simulink model "modele6git"  (R2024a)
settings: Solver=VariableStepAuto  StartTime=0.0  StopTime=20  RelTol=1e-6
values from neighbouring files (symbols this model uses):
  A_L = 1    [etablissement_variables.m]
  A_S = 3    [etablissement_variables.m]
  ampli_ent = 1    [etablissement_variables.m]
  C_x = 0.2    [etablissement_variables.m]
  Cte_1 = 10    [etablissement_variables.m]
  Cte_2 = 1.9    [etablissement_variables.m]
  Cte_3 = 1    [etablissement_variables.m]
  Cte_4 = 0.97    [etablissement_variables.m]
  d_f = 1    [etablissement_variables.m]
  d_r = 1    [etablissement_variables.m]
  EPSILON = 1e-9    (= 1e-09)    [etablissement_variables.m]
  f = 0.1    [etablissement_variables.m]
  freq_ent = 0.8    [etablissement_variables.m]
  g = 9.81    [etablissement_variables.m]
  h = 0.4    [etablissement_variables.m]
  Iz = 500    [etablissement_variables.m]
  J = mr/2*R.^2    [etablissement_variables.m]
  L = l_r+l_f    (= 2.9)    [etablissement_variables.m]
  l_f = 1.7    [etablissement_variables.m]
  l_r = 1.2    [etablissement_variables.m]
  M = 400    [etablissement_variables.m]
  R = [0.52 0.52 0.52 0.52]    [etablissement_variables.m]
  rho = 1    [etablissement_variables.m]
undefined symbols (not defined in the file or in its folder): angle_moy, calcul_adherence, calcul_delta, calcul_forceaero, calcul_forces, calcul_lambda, calcul_moteur, calcul_N, calcul_normevitesseroue, calcul_omega, calcul_retourvitesse, calcul_rotaroute, calcul_slipangle, calcul_vitessesroues, check_zeros_1, check_zeros_4, check_zeros_8, eqpfd, projection
libraries: simulink x8, cstblocks x4, spsTriangleGeneratorLib x3, embmathops x1, slpidlib x1
settings Model: SnapshotBufferSize=100  SnapshotInterval=1  Creator=TP-EEA  LastModifiedBy=TP-EEA
settings DebuggingCC: IgnoredZcDiagnostic=none

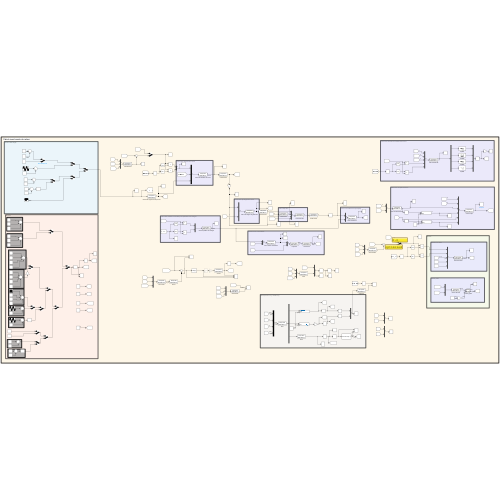
[thumbnail: Simulink's stored preview of the top-level diagram]
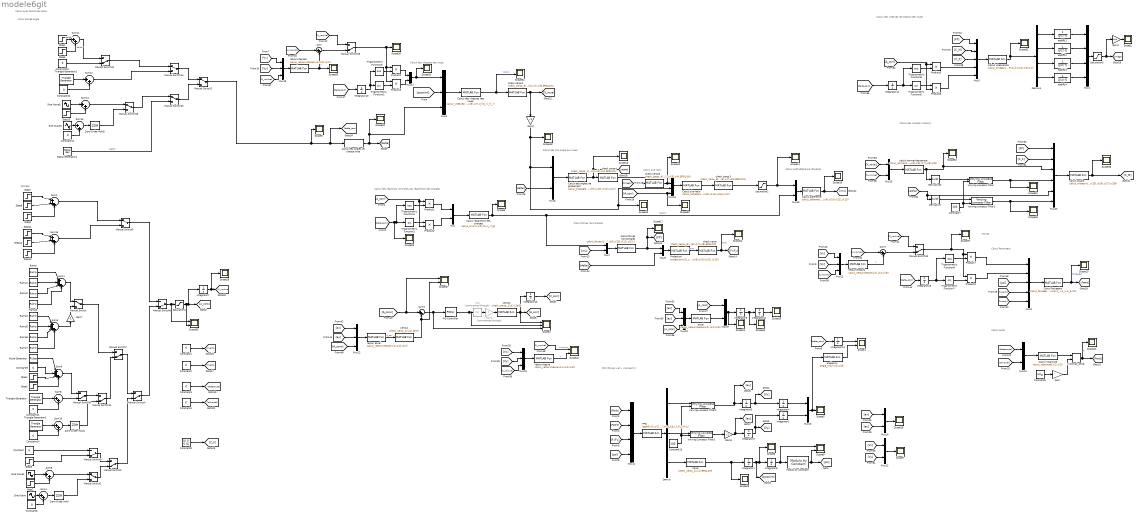
== system modele6git ==
  note: Calcul avec boucle de retour
  note: Calcul des vitesses des roues
  note: Entrées
  note: Choix entrée angle
  note: Calcul des vitesses de rotation des roues
  note: PFD (forces x et y, moment z)
  note: Calcul poids
  note: Calcul des slip-angle aux roues
  note: Calcul coef adhérence (Pacejka)
  note: Calcul slip-ratio
  note: Calcul des réactions normales par répartition des charges
  note: Calcul forces horizontales
  note: Forces
  note: Calcul force aéro
  note: Calcul des couples moteurs
  Abs : Abs  Commented=through  SaturateOnIntegerOverflow=off
  Calcul adhérence : MATLABFcn  MATLABFcn=calcul_adherence(u(1),u(2),u(3),u(4),u(5),u(6),u(7),u(8),Cte_1,Cte_2,Cte_3,Cte_4,u(9),u(10),u(11),u(12))  OutputDimensions=4*2
  Calcul des angles de chaque roue : MATLABFcn  MATLABFcn=calcul_delta(u,L,d_f)  OutputDimensions=4
  Calcul des angles de glissement : MATLABFcn  MATLABFcn=calcul_slipangle(u(1),u(2),u(3),u(4),u(5),u(6),u(7),u(8),u(9),u(10),u(11),u(12))  OutputDimensions=4
  Calcul des vitesses des roues : MATLABFcn  MATLABFcn=calcul_vitessesroues(u(1),u(2),u(3),u(4),u(5),u(6),u(7),d_f,d_r,l_f,l_r)  OutputDimensions=8
  Calcul forceaéro : MATLABFcn  MATLABFcn=calcul_forceaero(u(1),u(2),u(3),u(4),u(5),C_x,A_L,A_S,rho)  OutputDimensions=2
  Calcul forces horizontales : MATLABFcn  MATLABFcn=calcul_forces(u(1),u(2),u(3),u(4),u(5),u(6),u(7),u(8),u(9),u(10),u(11),u(12))  OutputDimensions=4*2
  Calcul rotaroute : MATLABFcn  MATLABFcn=calcul_rotaroute(u(1),u(2))  OutputDimensions=[3 3]  Output1D=off
  Calcul répartition des charges : MATLABFcn  MATLABFcn=calcul_N(u(1),u(2),M,L,l_r,h,g)  OutputDimensions=4
  Calcul slip-ratio : MATLABFcn  MATLABFcn=calcul_lambda(u(1),u(2),u(3),u(4),R(1),R(2),R(3),R(4),u(5),u(6),u(7),u(8),u(9),u(11),u(13),u(15),u(10),u(12),u(14),u(16),u(17))  OutputDimensions=4*2
  Calcul vitesserota : MATLABFcn  MATLABFcn=calcul_omega(u(1),u(2),u(3),u(4),u(5),u(6),u(7),u(8),u(9),u(10),u(11),u(12),u(13),u(14),u(15),u(16),u(17),u(18),R(1),R(2),R(3),R(4),J(1),J(2),J(3),J(4))  OutputDimensions=4
  Constant{,1..4,6,9..12,14..15} (12 alike) : Constant  Value=0
  Constant13 : Constant  Value=100  VectorParams1D=off
  Constant5 : Constant  Value=M*g  VectorParams1D=off
  Constant7 : Constant  Value=100  VectorParams1D=off
  Constant8 : Constant  Value=[0 0 0 0]
  Demux : Demux  Outputs=3
  Demux1 : Demux
  Derivative : Derivative
  Derivative2 : Derivative
  Gain : Gain  Gain=[0 0 1]'
  Gain1 : Gain  Gain=30/pi
  Gain2 : Gain  Gain=-1
  Gain3 : Gain  Gain=-1
  Gain7 : Gain  Gain=-1
  Gain8 : Gain  Commented=through  Gain=-1
  Integrator{1..7,9..15} (14 alike) : Integrator
  Manual Switch{,1..2,5,13..14,16} (7 alike) : ManualSwitch
  Manual Switch{3..4,6..12,15} (10 alike) : ManualSwitch  CurrentSetting=0
  Modulo by Constant : embmathops/Modulo by Constant  Denominator=2*pi  SimulateUsing=Code generation
      settings: LibrarySourceBlock=embeddedMathLib/Modulo by Constant
  Mux{,6..8,10,12..14,16..17,25,37} (12 alike) : Mux  Inputs=2
  Mux1 : Mux
  Mux11 : Mux
  Mux15 : Mux
  Mux{2,18..22} (6 alike) : Mux  Inputs=3
  Mux23 : Mux  Inputs=6
  Mux5 : Mux  Inputs=5
  Mux9 : Mux  Inputs=5
  PFD : MATLABFcn  MATLABFcn=eqpfd(u(1),u(2),u(4),u(5),u(6),u(7),u(8),u(9),u(10),u(11),u(12),u(13),u(14),d_f,d_r,l_f,l_r,M,Iz)  OutputDimensions=3
  PID Controller : slpidlib/PID Controller  Controller=PID  Form=Parallel  TimeDomain=Continuous-time  UseExternalTs=off  SampleTime=-1  IntegratorMethod=Forward Euler  FilterMethod=Forward Euler  ControllerParametersSource=internal  P=1.25  I=70  UseKiTs=off  D=0  UseExternalDerivativeSource=off  N=100  UseFilter=on  TunerSelectOption=Transfer Function Based (PID Tuner App)  InitialConditionSource=internal  InitialConditionForIntegrator=0  InitialConditionForFilter=0  DifferentiatorICPrevScaledInput=0  ExternalReset=none  TrackingMode=off  Kt=1  LimitOutput=off  SatLimitsSource=internal  UpperSaturationLimit=inf  LowerSaturationLimit=-inf  LinearizeAsGain=on  AntiWindupMode=none  Kb=1  LimitIntegrator=off  UpperIntegratorSaturationLimit=inf  LowerIntegratorSaturationLimit=-inf  POutMin=[]  POutMax=[]  IOutMin=[]  IOutMax=[]  DOutMin=[]  DOutMax=[]  NOutMin=[]  NOutMax=[]  SumOutMin=[]  SumOutMax=[]  SaturationOutMin=[]  SaturationOutMax=[]  PParamMin=[]  PParamMax=[]  IParamMin=[]  IParamMax=[]  DParamMin=[]  DParamMax=[]  NParamMin=[]  NParamMax=[]  KbParamMin=[]  KbParamMax=[]  KtParamMin=[]  KtParamMax=[]  KbOutMin=[]  KbOutMax=[]  KtOutMin=[]  KtOutMax=[]  IntegratorOutMin=[]  IntegratorOutMax=[]  FilterOutMin=[]  FilterOutMax=[]  SumI1OutMin=[]  SumI1OutMax=[]  SumI2OutMin=[]  SumI2OutMax=[]  SumI3OutMin=[]  SumI3OutMax=[]  SumI4OutMin=[]  SumI4OutMax=[]  SumDOutMin=[]  SumDOutMax=[]  DifferentiatorOutMin=[]  DifferentiatorOutMax=[]  FilterDiffOutCoefMin=[]  FilterDiffOutCoefMax=[]  ReciprocalOutMin=[]  ReciprocalOutMax=[]  SumDenOutMin=[]  SumDenOutMax=[]  SumNumOutMin=[]  SumNumOutMax=[]  DivideOutMin=[]  DivideOutMax=[]  UdiffTsProdOutMin=[]  UdiffTsProdOutMax=[]  NTsProdOutMin=[]  NTsProdOutMax=[]  UintegralTsProdOutMin=[]  UintegralTsProdOutMax=[]  UngainTsProdOutMin=[]  UngainTsProdOutMax=[]  ClampingZeroOutDataTypeStr=Inherit: Inherit via back propagation  ClampingZeroOutMin=[]  ClampingZeroOutMax=[]  FilterDenConstantOutDataTypeStr=Inherit: Inherit via back propagation  FilterDenConstantOutMin=[]  FilterDenConstantOutMax=[]  PCopyOutDataTypeStr=Inherit: Inherit via back propagation  PCopyOutMin=[]  PCopyOutMax=[]  NCopyOutDataTypeStr=Inherit: Inherit via back propagation  NCopyOutMin=[]  NCopyOutMax=[]  IntegratorContinuousStateAttributes=''  IntegratorStateMustResolveToSignalObject=off  IntegratorRTWStateStorageClass=Auto  FilterContinuousStateAttributes=''  FilterStateMustResolveToSignalObject=off  FilterRTWStateStorageClass=Auto  ParallelPVariant=InternalParameters  IdealPVariant=Disabled  IVariant=InternalParameters  DVariant=InternalParameters  IntegratorVariant=Continuous  SatVariant=Disabled  AWVariant=Passthrough  PCopyVariant=Disabled  TRVariant=Disabled  FdbkBlocksVariant=Forward  IdealPFdbkVariant=Disabled  SatFdbkVariant=Disabled  DerivativeFilterVariant=ContFilter  NVariant=InternalParameters  NCopyVariant=Disabled  FilterICVariant=InternalICsFilter  IntegratorICVariant=InternalICs  ExternalResetVariant=Disabled  TRSumVariant=Passthrough  SumFdbkVariant=Disabled  SumVariant=Sum_PID  TsampFilterVariant=InternalTs  TsampNgainVariant=Passthrough  TsampIntegralVariant=Disabled_SignalSpec  ExternalSaturationOutDataTypeStr=Inherit: Same as second input  DerivativeSourceVariant=ErrorSignal
  Product{1..8} (8 alike) : Product
  Projection : MATLABFcn  MATLABFcn=projection(u(1),u(2),u(3),u(4),u(5),u(6),u(7),u(8),u(9),u(10),u(11),u(12))  OutputDimensions=8
  Pulse Generator : DiscretePulseGenerator  PulseType=Time based  PulseWidth=56
  Ramp : simulink/Sources/Ramp  slope=1  start=0  InitialOutput=0.01
  Ramp1 : simulink/Sources/Ramp  slope=-1  start=3  InitialOutput=0
  Ramp2 : simulink/Sources/Ramp  slope=-1  start=7  InitialOutput=0
  Ramp3 : simulink/Sources/Ramp  slope=1  start=9  InitialOutput=0
  Ramp4 : simulink/Sources/Ramp  slope=1  start=0  InitialOutput=-0.01
  Ramp5 : simulink/Sources/Ramp  slope=-1  start=3  InitialOutput=0
  Ramp6 : simulink/Sources/Ramp  slope=-1  start=7  InitialOutput=0
  Ramp7 : simulink/Sources/Ramp  slope=1  start=9  InitialOutput=0
  Saturation1 : Saturate  UpperLimit=500  LowerLimit=0
  Saturation2 : Saturate  UpperLimit=100  LowerLimit=0
  Saturation3 : Saturate  UpperLimit=100000  LowerLimit=0
  Scope{1,9,22,27,33} (5 alike) : Scope  NumInputPorts=2
  Scope{2..3,5..8,10..21,23..26,28..30,32,34..37,49..52,54} (35 alike) : Scope
  Scope4 : Scope  NumInputPorts=3
  Signal Generator2 : SignalGenerator  Amplitude=0.2  Frequency=0.1  Units=rad/sec
  Sine Wave : Sin  Phase=pi/2  SampleTime=0
  Sine Wave1 : Sin  Amplitude=ampli_ent  Frequency=freq_ent  Phase=pi/1000  SampleTime=0
  Sine Wave2 : Sin  Amplitude=pi/2  Phase=pi/2  SampleTime=0
  Sine Wave3 : Sin  Amplitude=pi/2  Frequency=freq_ent  Phase=pi/1000  SampleTime=0
  Step1 : Step  After=pi/12  SampleTime=0
  Step10 : Step  Time=0  After=0  SampleTime=0
  Step11 : Step  Time=0  SampleTime=0
  Step12 : Step  Time=0.8  After=-1  SampleTime=0
  Step13 : Step  Time=1.75  SampleTime=0
  Step2 : Step  Time=0  After=0  SampleTime=0
  Step3 : Step  Time=2  After=-1  SampleTime=0
  Step4 : Step  Time=0.56*2  SampleTime=0
  Step5 : Step  Time=0  SampleTime=0
  Step6 : Step  Time=30  After=-pi/12  SampleTime=0
  Step7 : Step  Time=0  SampleTime=0
  Step8 : Step  After=-1  SampleTime=0
  Step9 : Step  Time=2  SampleTime=0
  Sum : Sum  Inputs=|+-
  Sum1 : Sum  Inputs=|++++
  Sum{4..5,8,10..14} (8 alike) : Sum  Inputs=|++
  Sum15 : Sum  Inputs=|+++
  Sum2 : Sum  Inputs=|+++
  Sum3 : Sum  Inputs=|+-
  Sum6 : Sum  Inputs=|++++
  Sum7 : Sum  Inputs=|+-
  Sum9 : Sum  Inputs=|++++
  Triangle Generator : spsTriangleGeneratorLib/Triangle Generator  Freq=1  Phase=90  Ts=0
  Triangle Generator1 : spsTriangleGeneratorLib/Triangle Generator  Freq=1  Phase=90  Ts=0
  Triangle Generator2 : spsTriangleGeneratorLib/Triangle Generator  Freq=1  Phase=90  Ts=0
  Trigonometric Function{1..2,5,7} (4 alike) : Trigonometry
  Trigonometric Function{3..4,6,8} (4 alike) : Trigonometry  Operator=cos
  Varying Lowpass Filter{,1..3} (4 alike) : cstblocks/Linear Parameter Varying/Varying Lowpass Filter  N=3
  Zero-Order Hold : ZeroOrderHold  SampleTime=0.1
  Zero-Order Hold1 : ZeroOrderHold  SampleTime=1/50
  Zero-Order Hold2 : ZeroOrderHold  SampleTime=0.1
  accel : MATLABFcn  MATLABFcn=calcul_retourvitesse(u(1),u(2),u(3))  OutputDimensions=1
  anglemoy : MATLABFcn  MATLABFcn=angle_moy(u(1),u(2))  OutputDimensions=1
  calcul couple : MATLABFcn  MATLABFcn=calcul_moteur(u(1),u(2),u(3),u(4),u(5),u(6),u(7),u(8),u(9),u(10),u(11),u(12),R(1),R(2),R(3),R(4),J(1),J(2),J(3),J(4),u(13),u(14),u(15),u(16),u(17),u(18),u(19),u(20),u(21),u(22),u(23),u(24),u(25),u(26),u(27),u(28))  OutputDimensions=4
  calcul normevitesseroue : MATLABFcn  MATLABFcn=calcul_normevitesseroue(u(1),u(2),u(3),u(4),u(5),u(6),u(7),u(8),u(9))  OutputDimensions=4
  check zeros : MATLABFcn  MATLABFcn=check_zeros_8(u(1),u(2),u(3),u(4),u(5),u(6),u(7),u(8),EPSILON)  OutputDimensions=8
  check zeros2 : MATLABFcn  MATLABFcn=check_zeros_8(u(1),u(2),u(3),u(4),u(5),u(6),u(7),u(8),EPSILON)  OutputDimensions=8
  check zeros3 : MATLABFcn  MATLABFcn=check_zeros_8(u(1),u(2),u(3),u(4),u(5),u(6),u(7),u(8),EPSILON)  OutputDimensions=8
  check zeros4 : MATLABFcn  MATLABFcn=check_zeros_4(u(1),u(2),u(3),u(4),EPSILON)  OutputDimensions=4
  check zeros5 : MATLABFcn  MATLABFcn=check_zeros_4(u(1),u(2),u(3),u(4),EPSILON)  OutputDimensions=4
  eqdiffz1 : TransferFcn  Denominator=[J(1) f]
  eqdiffz2 : TransferFcn  Denominator=[J(2) f]
  eqdiffz3 : TransferFcn  Denominator=[J(3) f]
  eqdiffz4 : TransferFcn  Denominator=[J(4) f]
  multmat_poids : Product  Multiplication=Matrix(*)
  retour accel : MATLABFcn  MATLABFcn=calcul_retourvitesse(u(1),u(2),u(3))  OutputDimensions=1
  retourvitesse : MATLABFcn  MATLABFcn=calcul_retourvitesse(u(1),u(2),u(3))  OutputDimensions=1
  retourvitesse1 : MATLABFcn  MATLABFcn=calcul_retourvitesse(u(1),u(2),u(3))  OutputDimensions=1
  retourvitesse2 : MATLABFcn  MATLABFcn=calcul_retourvitesse(u(1),u(2),u(3))  OutputDimensions=1
  zeros : MATLABFcn  MATLABFcn=check_zeros_1(u(1),EPSILON)
  zeros1 : MATLABFcn  MATLABFcn=check_zeros_1(u(1),1e-9)
  zeros2 : MATLABFcn  MATLABFcn=check_zeros_1(u(1),1e-9)
  wires:
  Calcul des angles de glissement/1 -> check zeros4/1, [alpha], Scope13/1
  Mux17/1 -> Scope20/1, Mux2/1
  [Vventy] -> Mux9/5
  [ay] -> Mux22/2
  [ax] -> Mux22/1
  Mux9/1 -> Calcul forceaéro/1
  Mux2/1 -> Calcul des vitesses des roues/1
  Calcul adhérence/1 -> Scope16/1, [mu]
  [A_cons] -> Sum3/1, Scope27/1
  Mux22/1 -> retour accel/1
  [thetaroute] -> Mux10/1
  [Vx] -> Mux20/1
  eqdiffz4/1 -> Mux1/4
  [Faero] -> Mux11/2
  retourvitesse/1 -> Scope22/2  "V"
  [ax] -> Mux19/1
  Mux11/1 -> PFD/1
  [Poids] -> Mux11/1
  Manual Switch2/1 -> [delta_com], Calcul des angles de chaque roue/1, Scope5/1
  Trigonometric Function3/1 -> Product2/2
  Product2/1 -> Mux17/1
  Projection/1 -> check zeros/1  "FxFy"
  Trigonometric Function2/1 -> Product3/2
  [A_corr] -> Scope30/1, Mux15/4
  PFD/1 -> Demux/1
  Mux8/1 -> Projection/1
  Constant5/1 -> Gain/1
  Mux6/1 -> Calcul des angles de glissement/1
  Integrator2/1 -> Mux13/2
  Mux7/1 -> Calcul forces horizontales/1
  multmat_poids/1 -> Scope11/1, [Poids]  "P"
  Product3/1 -> Mux17/2
  Mux10/1 -> Calcul rotaroute/1
  Calcul forceaéro/1 -> Scope10/1, [Faero]  "forceaéro"
  Integrator1/1 -> Scope8/1, Integrator6/1, [psipoint]
  Mux15/1 -> Calcul slip-ratio/1
  [FxFy] -> Mux11/3
  [delta_com] -> Integrator10/1
  Gain/1 -> multmat_poids/2
  Mux20/1 -> retourvitesse/1
  [mu] -> Mux7/2
  Mux14/1 -> Scope15/1
  [psipoint] -> Mux2/2
  Integrator4/1 -> Mux13/1
  [Vventx] -> Mux9/4
  [psi] -> Mux9/3
  [ax] -> Mux14/1
  [ay] -> Mux14/2
  Mux12/1 -> Scope7/1
  Integrator5/1 -> [Vx], Integrator4/1
  [phiroute] -> Mux10/2
  Integrator6/1 -> Modulo by Constant/1, Scope9/1
  [Vx] -> Mux12/1
  Mux13/1 -> anglemoy/1, Scope3/1
  eqdiffz3/1 -> Mux1/3
  calcul couple/1 -> Scope36/1, [C_M]
  [Vy] -> Mux12/2
  Calcul rotaroute/1 -> multmat_poids/1
  Constant1/1 -> [Vventx]
  Calcul des angles de chaque roue/1 -> [delta], Mux2/3, Scope18/1
  Calcul répartition des charges/1 -> Mux16/2, Mux7/1, Scope6/1  "N_cons"
  Constant4/1 -> [phiroute]
  Constant2/1 -> [Vventy]
  Integrator3/1 -> Integrator2/1, [Vy]
  Demux1/4 -> eqdiffz4/1
  Constant8/1 -> [C_F]
  eqdiffz2/1 -> Mux1/2
  [C_M] -> Mux5/2
  Mux19/1 -> accel/1
  Mux5/1 -> Calcul vitesserota/1
  Calcul vitesserota/1 -> Scope32/1, Demux1/1
  [delta] -> Mux8/2
  retour accel/1 -> zeros1/1  "A_ret"
  Mux1/1 -> Saturation3/1
  [C_F] -> Mux5/3
  eqdiffz1/1 -> Mux1/1
  Constant3/1 -> [thetaroute]
  Demux1/3 -> eqdiffz3/1
  Demux1/2 -> eqdiffz2/1
  Demux1/1 -> eqdiffz1/1
  Product4/1 -> Mux/2
  [ay] -> Mux19/2
  [Vy] -> Mux20/2
  Modulo by Constant/1 -> [psi], Scope9/2
  Manual Switch6/1 -> Saturation1/1, Scope33/1
  Manual Switch1/1 -> Manual Switch3/2
  Zero-Order Hold/1 -> Manual Switch1/2
  Gain1/1 -> Scope2/1
  [omega] -> check zeros5/1
  [FP] -> Mux5/1
  [V_voulue] -> Scope22/1  "Vvoulue"
  zeros/1 -> Scope29/1, Integrator1/1
  [Vy] -> Mux18/2
  [Vx] -> Mux18/1
  [V_voulue] -> Sum/1
  retourvitesse2/1 -> Sum/2, Scope50/1  "V"
  Mux18/1 -> retourvitesse2/1
  [psi] -> Mux11/4
  [delta] -> Mux6/2
  Calcul forces horizontales/1 -> Scope17/1, [FP], Mux8/1
  Mux/1 -> Calcul répartition des charges/1
  Calcul des vitesses des roues/1 -> Scope54/1, check zeros2/1  "Vrcons"
  [FP] -> Mux23/1
  [C_F] -> Mux23/2
  Mux23/1 -> calcul couple/1
  check zeros/1 -> Scope12/1, [FxFy]  "FxFy"
  Ramp/1 -> Sum1/1
  Ramp1/1 -> Sum1/2
  Ramp2/1 -> Sum1/3
  Ramp3/1 -> Sum1/4
  Integrator7/1 -> [V_voulue], Scope28/1
  Trigonometric Function1/1 -> Product4/1
  Product1/1 -> Mux/1
  Trigonometric Function4/1 -> Product1/2
  Product5/1 -> Mux5/4
  [delta_com] -> Integrator11/1
  [A_corr] -> Product5/1, Product6/2
  Product6/1 -> Mux5/5
  Trigonometric Function6/1 -> Product5/2
  Trigonometric Function5/1 -> Product6/1
  Sine Wave/1 -> Sum4/1
  Sum4/1 -> Zero-Order Hold/1
  Constant6/1 -> Sum4/2
  Sum5/1 -> Manual Switch1/1
  Sine Wave1/1 -> Sum5/1
  Step2/1 -> Sum5/2
  Integrator12/1 -> Scope35/1
  Mux21/1 -> retourvitesse1/1
  Manual Switch10/1 -> Scope37/1, Product8/1, Product7/1
  Product7/1 -> Mux9/1
  Product8/1 -> Mux9/2
  [Vx] -> Mux21/1
  [delta_com] -> Integrator13/1
  Trigonometric Function7/1 -> Product8/2
  [V_voulue] -> Sum7/1
  [Vy] -> Mux21/2
  retourvitesse1/1 -> Sum7/2  "V"
  Trigonometric Function8/1 -> Product7/2
  [A_cons] -> Mux22/3
  [A_cons] -> Mux19/3
  [V_voulue] -> Mux18/3
  [V_voulue] -> Mux21/3
  [V_voulue] -> Mux20/3
  [alpha] -> Derivative/1, Mux23/5
  calcul normevitesseroue/1 -> Scope52/1, Mux23/3, Derivative2/1
  Mux25/1 -> calcul normevitesseroue/1
  [V_roue] -> Mux25/1
  [V_voulue] -> Mux25/2
  Sum1/1 -> Manual Switch/1
  Abs/1 -> Gain8/1
  Demux/3 -> zeros/1
  Calcul slip-ratio/1 -> check zeros3/1
  Mux16/1 -> Calcul adhérence/1
  zeros1/1 -> Sum3/2, Scope27/2
  zeros2/1 -> Integrator15/1, Scope4/1, [A_corr]
  Varying Lowpass Filter1/1 -> Scope49/1, Mux23/6
  Gain8/1 -> zeros2/1
  Manual Switch15/1 -> Product3/1, Product2/1, Scope26/1
  Ramp7/1 -> Sum6/4
  Ramp5/1 -> Sum6/2
  Sum6/1 -> Gain7/1
  Ramp6/1 -> Sum6/3
  Ramp4/1 -> Sum6/1
  Gain7/1 -> Manual Switch/2
  Manual Switch/1 -> Manual Switch7/1
  Pulse Generator/1 -> Sum9/1
  Constant9/1 -> Sum9/2
  Step4/1 -> Sum9/3
  Step3/1 -> Sum9/4
  Saturation1/1 -> Scope33/2, [A_cons], Integrator7/1
  Sum9/1 -> Manual Switch8/1
  Sum8/1 -> Manual Switch8/2
  Triangle Generator/1 -> Sum8/1
  Constant11/1 -> Sum8/2
  [A_cons] -> Mux37/1
  Mux37/1 -> Scope21/1, Integrator9/1
  accel/1 -> Mux37/2
  Integrator9/1 -> Scope34/1, Integrator12/1
  Manual Switch9/1 -> Manual Switch3/1
  Constant/1 -> Manual Switch9/1
  Step5/1 -> Manual Switch9/2
  Sum10/1 -> Zero-Order Hold1/1
  Constant14/1 -> Sum10/2
  Triangle Generator1/1 -> Sum10/1
  Zero-Order Hold1/1 -> Manual Switch11/2
  Manual Switch8/1 -> Manual Switch11/1
  Manual Switch11/1 -> Manual Switch7/2
  Step1/1 -> Sum11/1  "delta*"
  Step6/1 -> Sum11/2  "delta*"
  Sum11/1 -> Manual Switch12/1
  Constant15/1 -> Manual Switch12/2
  Saturation2/1 -> Mux16/1, Scope14/1
  [delta_com] -> Scope23/1, Trigonometric Function4/1, Trigonometric Function1/1
  Gain3/1 -> Integrator3/1, [ay]
  Varying Lowpass Filter3/1 -> [ax], Integrator5/1
  check zeros3/1 -> Saturation2/1
  Integrator10/1 -> Trigonometric Function3/1, Trigonometric Function2/1
  Integrator11/1 -> Trigonometric Function6/1, Trigonometric Function5/1
  Integrator13/1 -> Trigonometric Function8/1, Trigonometric Function7/1
  Derivative2/1 -> Varying Lowpass Filter/1
  Varying Lowpass Filter/1 -> Scope51/1, Mux23/4
  Derivative/1 -> Varying Lowpass Filter1/1
  Constant7/1 -> Varying Lowpass Filter1/2, Varying Lowpass Filter/2
  Manual Switch3/1 -> Manual Switch4/2
  Manual Switch7/1 -> Manual Switch4/1
  Manual Switch4/1 -> Manual Switch6/2
  Manual Switch5/1 -> Manual Switch6/1
  Step7/1 -> Sum2/1
  Step8/1 -> Sum2/2
  Step9/1 -> Sum2/3
  Sum2/1 -> Manual Switch5/1
  Sum12/1 -> Manual Switch14/2
  Triangle Generator2/1 -> Sum12/1
  Constant10/1 -> Sum12/2
  Step10/1 -> Sum14/2
  Zero-Order Hold2/1 -> Manual Switch16/2
  Sum13/1 -> Zero-Order Hold2/1
  Sum14/1 -> Manual Switch16/1
  Sine Wave3/1 -> Sum14/1
  Constant12/1 -> Sum13/2
  Sine Wave2/1 -> Sum13/1
  Manual Switch14/1 -> Manual Switch2/1
  Manual Switch13/1 -> Manual Switch2/2
  Signal Generator2/1 -> Manual Switch13/2  "delta*"
  Manual Switch16/1 -> Manual Switch13/1
  Manual Switch12/1 -> Manual Switch14/1
  Sum15/1 -> Manual Switch5/2
  Step12/1 -> Sum15/2
  Step11/1 -> Sum15/1
  Step13/1 -> Sum15/3
  [delta_com] -> Integrator14/1
  anglemoy/1 -> Scope1/2
  Saturation3/1 -> [omega], Gain1/1
  Demux/2 -> Varying Lowpass Filter2/1
  Varying Lowpass Filter2/1 -> Gain3/1
  Demux/1 -> Varying Lowpass Filter3/1
  Constant13/1 -> Varying Lowpass Filter3/2, Varying Lowpass Filter2/2
  Integrator14/1 -> Scope1/1
  Integrator15/1 -> [V_corr]
  Sum7/1 -> Manual Switch10/2
  [V_voulue] -> Manual Switch10/1
  [V_voulue] -> Manual Switch15/1
  Sum/1 -> Manual Switch15/2
  PID Controller/1 -> Scope4/2, Abs/1
  Sum3/1 -> PID Controller/1, Scope4/3
  [A_corr] -> Product1/1, Product4/2
  check zeros2/1 -> Gain2/1, [V_roue]
  check zeros4/1 -> Mux15/1
  check zeros5/1 -> Scope24/1, Mux15/2
  Gain2/1 -> Mux6/1, Mux15/3, Scope25/1, Scope19/1
